simulink model "fft32kpt_ssr32_float"  (R2024a)
settings: Solver=VariableStepAuto  StartTime=0.0  StopTime=sample_period*N*6  RelTol=1e-3
PreLoadFcn:
  | clk_freq = 570e6;
  | SSR=32; % transpose block SSR settings...
  | sample_period = 1/(SSR*clk_freq);
  | N=32768; % fft point size
  | binw=(1/sample_period) / (2*N); % bin width
  | bin_freq = 2*pi*3*binw+pi*binw; % sin, cos freq centered in channel
  | 
  | % for transpose block
  | DATA_WIDTH=32;
  | M=32;
  | N1=N/M;
  | MEM_STYLE=4; % MEM OPTIONS: 4 - ULTRA, 0 - AUTO, 1 - BRAM, 5 - MIXED
InitFcn:
  | clk_freq = 570e6;
  | SSR=32; % transpose block SSR settings...
  | sample_period = 1/(SSR*clk_freq);
  | N=32768; % fft point size
  | binw=(1/sample_period) / (2*N); % bin width
  | bin_freq = 2*pi*3*binw+pi*binw; % sin, cos freq centered in channel
  | 
  | % for transpose block
  | DATA_WIDTH=32;
  | M=32;
  | N1=N/M;
  | MEM_STYLE=4; % MEM OPTIONS: 4 - ULTRA, 0 - AUTO, 1 - BRAM, 5 - MIXED
undefined symbols (not defined in the file or in its folder): None, S, vsva2197, xcvc1902
libraries: hdlBasic x139, aieBasic x95, aieUtilities x32, aieDSP x32, hdlUtilities x32, matrix_library x32, hdlSSR x12, hdlDSPIP x1, simulink x1, dspxfrm3 x1, vmcUtilities x1
(part 3 of 4)

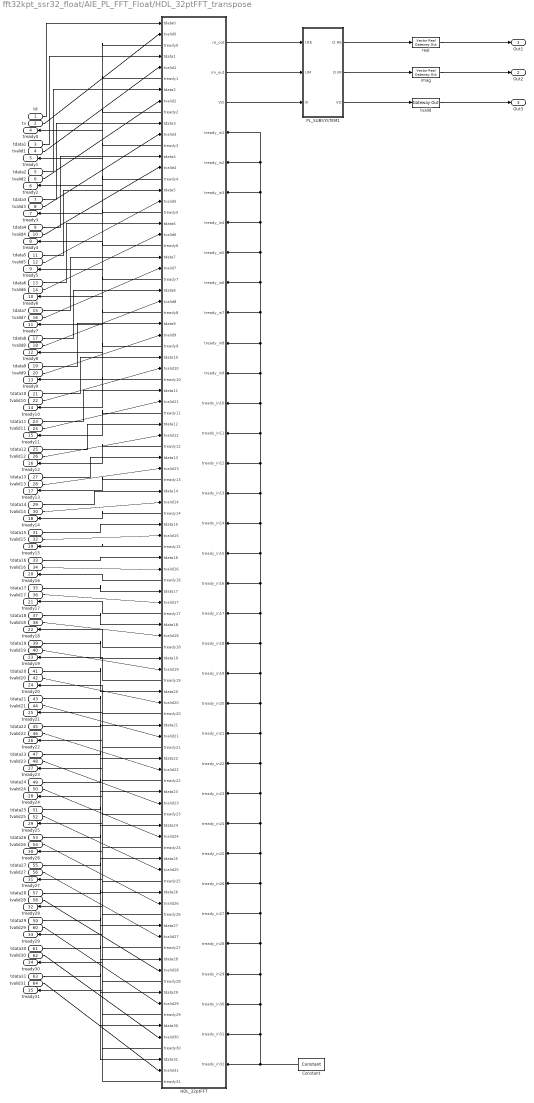
== system fft32kpt_ssr32_float/AIE_PL_FFT_Float/HDL_32ptFFT_transpose ==
  td : Inport
  tv : Inport  Port=2
  tdata1 : Inport  Port=3
  tvalid1 : Inport  Port=4
  tdata2 : Inport  Port=5
  tvalid2 : Inport  Port=6
  tdata3 : Inport  Port=7
  tvalid3 : Inport  Port=8
  tdata4 : Inport  Port=9
  tvalid4 : Inport  Port=10
  tdata5 : Inport  Port=11
  tvalid5 : Inport  Port=12
  tdata6 : Inport  Port=13
  tvalid6 : Inport  Port=14
  tdata7 : Inport  Port=15
  tvalid7 : Inport  Port=16
  tdata8 : Inport  Port=17
  tvalid8 : Inport  Port=18
  tdata9 : Inport  Port=19
  tvalid9 : Inport  Port=20
  tdata10 : Inport  Port=21
  tvalid10 : Inport  Port=22
  tdata11 : Inport  Port=23
  tvalid11 : Inport  Port=24
  tdata12 : Inport  Port=25
  tvalid12 : Inport  Port=26
  tdata13 : Inport  Port=27
  tvalid13 : Inport  Port=28
  tdata14 : Inport  Port=29
  tvalid14 : Inport  Port=30
  tdata15 : Inport  Port=31
  tvalid15 : Inport  Port=32
  tdata16 : Inport  Port=33
  tvalid16 : Inport  Port=34
  tdata17 : Inport  Port=35
  tvalid17 : Inport  Port=36
  tdata18 : Inport  Port=37
  tvalid18 : Inport  Port=38
  tdata19 : Inport  Port=39
  tvalid19 : Inport  Port=40
  tdata20 : Inport  Port=41
  tvalid20 : Inport  Port=42
  tdata21 : Inport  Port=43
  tvalid21 : Inport  Port=44
  tdata22 : Inport  Port=45
  tvalid22 : Inport  Port=46
  tdata23 : Inport  Port=47
  tvalid23 : Inport  Port=48
  tdata24 : Inport  Port=49
  tvalid24 : Inport  Port=50
  tdata25 : Inport  Port=51
  tvalid25 : Inport  Port=52
  tdata26 : Inport  Port=53
  tvalid26 : Inport  Port=54
  tdata27 : Inport  Port=55
  tvalid27 : Inport  Port=56
  tdata28 : Inport  Port=57
  tvalid28 : Inport  Port=58
  tdata29 : Inport  Port=59
  tvalid29 : Inport  Port=60
  tdata30 : Inport  Port=61
  tvalid30 : Inport  Port=62
  tdata31 : Inport  Port=63
  tvalid31 : Inport  Port=64
  Constant : hdlBasic/Constant  const=1.0  gui_display_data_type=Boolean  arith_type=Boolean  n_bits=16  bin_pt=14  preci_type=Single  exp_width=8  frac_width=24  explicit_period=on  period=1/clk_freq  XmcBlockStatus=1  maskContainerNames=tabcontainer1  block_type=constant  block_config=sysgen:Constant_config
  HDL_32ptFFT : Subsystem
      settings: PortSchema="{\"entries\":[{\"content\":{\"sides\":[{\"content\":{\"connectorIds\":[\"In1\",\"In2\",\"Out4\",\"In3\",\"In4\",\"Out5\",\"In5\",\"In6\",\"Out6\",\"In7\",\"In8\",\"Out7\",\"In9\",\"In10\",\"Out8\",\"In11\",\"In12\",\"Out9\",\"In13\",\"In14\",\"Out10\",\"In15\",\"In16\",\"Out11\",\"In17\",\"In18\",\"Out12\",\"In19\",\"In20\",\"Out13\",\"In21\",\"In22\",\"Out14\",\"In23\",\"In24\",\"Out15\",\"In25\",\"In26\",\"Out16\",\"In27\",\"In28\",\"Out17\",\"In29\",\"In30\",\"Out18\",\"In31\",\"In32\",\"Out19\",\"In33\",\"In34\",\"Out20\",\"In35\",\"In36\",\"Out21\",\"In37\",\"In38\",\"Out22\",\"In39\",\"In40\",\"Out23\",\"In41\",\"In42\",\"Out24\",\"In43\",\"In44\",\"Out25\",\"In45\",\"In46\",\"Out26\",\"In47\",\"In48\",\"Out27\",\"In49\",\"In50\",\"Out28\",\"In51\",\"In52\",\"Out29\",\"In53\",\"In54\",\"Out30\",\"In55\",\"In56\",\"Out31\",\"In57\",\"In58\",\"Out32\",\"In59\",\"In60\",\"Out33\",\"In61\",\"In62\",\"Out34\",\"In63\",\"In64\",\"Out35\"]},\"type\":\"ConnectorPlacement.EquallySpacedRectSide\",\"uuid\":\"a3725b6b-e4a3-4f45-ab24-220566ddd85d\"},{\"content\":{\"connectorIds\":[\"Out1\",\"Out2\",\"Out3\",\"In65\",\"In66\",\"In67\",\"In68\",\"In69\",\"In70\",\"In71\",\"In72\",\"In73\",\"In74\",\"In75\",\"In76\",\"In77\",\"In78\",\"In79\",\"In80\",\"In81\",\"In82\",\"In83\",\"In84\",\"In85\",\"In86\",\"In87\",\"In88\",\"In89\",\"In90\",\"In91\",\"In92\",\"In93\",\"In94\",\"In95\",\"In96\"],\"side\":\"RIGHT\"},\"type\":\"ConnectorPlacement.EquallySpacedRectSide\",\"uuid\":\"6d1cacb8-7866-41d1-bf7d-cacacc53b5ea\"},{\"content\":{\"side\":\"TOP\"},\"type\":\"ConnectorPlacement.EquallySpacedRectSide\",\"uuid\":\"e352e270-c6f1-4bf3-b401-eafc9b9ac14e\"},{\"content\":{\"side\":\"BOTTOM\"},\"type\":\"ConnectorPlacement.EquallySpacedRectSide\",\"uuid\":\"85cad029-9e0a-42ad-b7dd-28c8d75053c6\"}]},\"type\":\"ConnectorPlacement.EquallySpacedConnector\",\"uuid\":\"92e4a087-3b5f-44ab-84c8-8a9b01a0fbf2\"}],\"packageUris\":[\"http://schema.mathworks.com/mf0/Connector/R2020b\"],\"version\":\"1.0\"}"
  PL_SUBSYSTEM1 : Subsystem
  imag : hdlSSR/Vector Real Gateway Out  inherit_from_input=on  hdl_port=on  sg_ssr=32  rows=1  columns=1  UseAsDAC=off  DACChannel='1'  interface=None  automatic_assignment=on  address_offset=hex2dec('00')  intf_name=''  intf_description=''  timing_constraint=None  locs_specified=off  LOCs={}  io_standard={}  block_type=realgatewayout_ssr  XmcBlockStatus=1  sg_ssr_prev=32  maskContainerNames=group4  block_width_w=590  block_height_w=620  block_width=620  block_height=750
  real : hdlSSR/Vector Real Gateway Out  inherit_from_input=on  hdl_port=on  sg_ssr=32  rows=1  columns=1  UseAsDAC=off  DACChannel='1'  interface=None  automatic_assignment=on  address_offset=hex2dec('00')  intf_name=''  intf_description=''  timing_constraint=None  locs_specified=off  LOCs={}  io_standard={}  block_type=realgatewayout_ssr  XmcBlockStatus=1  sg_ssr_prev=32  maskContainerNames=group4  block_width_w=590  block_height_w=620  block_width=620  block_height=750
  tvalid : hdlBasic/Gateway Out  inherit_from_input=on  bool_to_boolean=off  hdl_port=on  rows=1  columns=1  UseAsDAC=off  DACChannel='1'  interface=None  automatic_assignment=on  address_offset=hex2dec('00')  intf_name=''  intf_description=''  timing_constraint=None  locs_specified=off  LOCs={}  io_standard={}  XmcBlockStatus=1  maskContainerNames=group4  block_type=gatewayout  block_config=sysgen:gateway_out_config  block_width_w=590  block_height_w=620  block_width=620  block_height=750
  Out1 : Outport
  Out2 : Outport  Port=2
  Out3 : Outport  Port=3
  tready0 : Outport  Port=4
  tready1 : Outport  Port=5
  tready2 : Outport  Port=6
  tready3 : Outport  Port=7
  tready4 : Outport  Port=8
  tready5 : Outport  Port=9
  tready6 : Outport  Port=10
  tready7 : Outport  Port=11
  tready8 : Outport  Port=12
  tready9 : Outport  Port=13
  tready10 : Outport  Port=14
  tready11 : Outport  Port=15
  tready12 : Outport  Port=16
  tready13 : Outport  Port=17
  tready14 : Outport  Port=18
  tready15 : Outport  Port=19
  tready16 : Outport  Port=20
  tready17 : Outport  Port=21
  tready18 : Outport  Port=22
  tready19 : Outport  Port=23
  tready20 : Outport  Port=24
  tready21 : Outport  Port=25
  tready22 : Outport  Port=26
  tready23 : Outport  Port=27
  tready24 : Outport  Port=28
  tready25 : Outport  Port=29
  tready26 : Outport  Port=30
  tready27 : Outport  Port=31
  tready28 : Outport  Port=32
  tready29 : Outport  Port=33
  tready30 : Outport  Port=34
  tready31 : Outport  Port=35
  wires:
  HDL_32ptFFT/16(tready12) -> tready12/1
  tdata23/1 -> HDL_32ptFFT/47(tdata23)
  tdata17/1 -> HDL_32ptFFT/35(tdata17)
  HDL_32ptFFT/22(tready18) -> tready18/1
  tdata6/1 -> HDL_32ptFFT/13(tdata6)
  HDL_32ptFFT/17(tready13) -> tready13/1
  tvalid26/1 -> HDL_32ptFFT/54(tvalid26)
  HDL_32ptFFT/8(tready4) -> tready4/1
  tv/1 -> HDL_32ptFFT/2(tvalid0)
  HDL_32ptFFT/31(tready27) -> tready27/1
  tvalid11/1 -> HDL_32ptFFT/24(tvalid11)
  real/1 -> Out1/1
  tvalid27/1 -> HDL_32ptFFT/56(tvalid27)
  HDL_32ptFFT/34(tready30) -> tready30/1
  tdata10/1 -> HDL_32ptFFT/21(tdata10)
  tvalid6/1 -> HDL_32ptFFT/14(tvalid6)
  HDL_32ptFFT/5(tready1) -> tready1/1
  tvalid3/1 -> HDL_32ptFFT/8(tvalid3)
  tvalid22/1 -> HDL_32ptFFT/46(tvalid22)
  HDL_32ptFFT/32(tready28) -> tready28/1
  tvalid4/1 -> HDL_32ptFFT/10(tvalid4)
  HDL_32ptFFT/30(tready26) -> tready26/1
  tdata1/1 -> HDL_32ptFFT/3(tdata1)
  tdata28/1 -> HDL_32ptFFT/57(tdata28)
  tdata5/1 -> HDL_32ptFFT/11(tdata5)
  HDL_32ptFFT/12(tready8) -> tready8/1
  HDL_32ptFFT/15(tready11) -> tready11/1
  tvalid31/1 -> HDL_32ptFFT/64(tvalid31)
  tdata25/1 -> HDL_32ptFFT/51(tdata25)
  tvalid25/1 -> HDL_32ptFFT/52(tvalid25)
  tvalid29/1 -> HDL_32ptFFT/60(tvalid29)
  HDL_32ptFFT/35(tready31) -> tready31/1
  tvalid2/1 -> HDL_32ptFFT/6(tvalid2)
  HDL_32ptFFT/28(tready24) -> tready24/1
  HDL_32ptFFT/13(tready9) -> tready9/1
  PL_SUBSYSTEM1/1(O.RE) -> real/1
  HDL_32ptFFT/18(tready14) -> tready14/1
  tdata27/1 -> HDL_32ptFFT/55(tdata27)
  tdata16/1 -> HDL_32ptFFT/33(tdata16)
  tdata12/1 -> HDL_32ptFFT/25(tdata12)
  tvalid18/1 -> HDL_32ptFFT/38(tvalid18)
  tdata4/1 -> HDL_32ptFFT/9(tdata4)
  tvalid16/1 -> HDL_32ptFFT/34(tvalid16)
  tdata13/1 -> HDL_32ptFFT/27(tdata13)
  imag/1 -> Out2/1
  HDL_32ptFFT/4(tready0) -> tready0/1
  tvalid28/1 -> HDL_32ptFFT/58(tvalid28)
  HDL_32ptFFT/9(tready5) -> tready5/1
  tdata18/1 -> HDL_32ptFFT/37(tdata18)
  HDL_32ptFFT/21(tready17) -> tready17/1
  tdata26/1 -> HDL_32ptFFT/53(tdata26)
  HDL_32ptFFT/6(tready2) -> tready2/1
  tdata29/1 -> HDL_32ptFFT/59(tdata29)
  tdata15/1 -> HDL_32ptFFT/31(tdata15)
  tdata11/1 -> HDL_32ptFFT/23(tdata11)
  Constant/1 -> HDL_32ptFFT/94(tready_in30), HDL_32ptFFT/93(tready_in29), HDL_32ptFFT/92(tready_in28), HDL_32ptFFT/91(tready_in27), HDL_32ptFFT/90(tready_in26), HDL_32ptFFT/89(tready_in25), HDL_32ptFFT/88(tready_in24), HDL_32ptFFT/87(tready_in23), HDL_32ptFFT/86(tready_in22), HDL_32ptFFT/85(tready_in21), HDL_32ptFFT/84(tready_in20), HDL_32ptFFT/83(tready_in19), HDL_32ptFFT/82(tready_in18), HDL_32ptFFT/81(tready_in17), HDL_32ptFFT/80(tready_in16), HDL_32ptFFT/79(tready_in15), HDL_32ptFFT/78(tready_in14), HDL_32ptFFT/77(tready_in13), HDL_32ptFFT/76(tready_in12), HDL_32ptFFT/75(tready_in11), HDL_32ptFFT/74(tready_in10), HDL_32ptFFT/73(tready_in9), HDL_32ptFFT/72(tready_in8), HDL_32ptFFT/71(tready_in7), HDL_32ptFFT/69(tready_in5), HDL_32ptFFT/68(tready_in4), HDL_32ptFFT/67(tready_in3), HDL_32ptFFT/66(tready_in2), HDL_32ptFFT/65(tready_in1), HDL_32ptFFT/70(tready_in6), HDL_32ptFFT/95(tready_in31), HDL_32ptFFT/96(tready_in32)
  tvalid23/1 -> HDL_32ptFFT/48(tvalid23)
  HDL_32ptFFT/19(tready15) -> tready15/1
  tdata19/1 -> HDL_32ptFFT/39(tdata19)
  tvalid14/1 -> HDL_32ptFFT/30(tvalid14)
  HDL_32ptFFT/10(tready6) -> tready6/1
  HDL_32ptFFT/23(tready19) -> tready19/1
  tvalid1/1 -> HDL_32ptFFT/4(tvalid1)
  tvalid10/1 -> HDL_32ptFFT/22(tvalid10)
  HDL_32ptFFT/27(tready23) -> tready23/1
  tdata9/1 -> HDL_32ptFFT/19(tdata9)
  tvalid12/1 -> HDL_32ptFFT/26(tvalid12)
  tvalid13/1 -> HDL_32ptFFT/28(tvalid13)
  HDL_32ptFFT/7(tready3) -> tready3/1
  tvalid21/1 -> HDL_32ptFFT/44(tvalid21)
  tvalid15/1 -> HDL_32ptFFT/32(tvalid15)
  tdata8/1 -> HDL_32ptFFT/17(tdata8)
  tdata20/1 -> HDL_32ptFFT/41(tdata20)
  tdata24/1 -> HDL_32ptFFT/49(tdata24)
  tvalid24/1 -> HDL_32ptFFT/50(tvalid24)
  PL_SUBSYSTEM1/3(VO) -> tvalid/1
  tvalid20/1 -> HDL_32ptFFT/42(tvalid20)
  tdata21/1 -> HDL_32ptFFT/43(tdata21)
  tdata30/1 -> HDL_32ptFFT/61(tdata30)
  tdata2/1 -> HDL_32ptFFT/5(tdata2)
  HDL_32ptFFT/11(tready7) -> tready7/1
  HDL_32ptFFT/33(tready29) -> tready29/1
  HDL_32ptFFT/24(tready20) -> tready20/1
  HDL_32ptFFT/25(tready21) -> tready21/1
  tdata3/1 -> HDL_32ptFFT/7(tdata3)
  tvalid19/1 -> HDL_32ptFFT/40(tvalid19)
  tdata31/1 -> HDL_32ptFFT/63(tdata31)
  tdata14/1 -> HDL_32ptFFT/29(tdata14)
  HDL_32ptFFT/20(tready16) -> tready16/1
  HDL_32ptFFT/3(VO) -> PL_SUBSYSTEM1/3(VI)
  HDL_32ptFFT/1(re_out) -> PL_SUBSYSTEM1/1(I.RE)
  tdata7/1 -> HDL_32ptFFT/15(tdata7)
  tvalid/1 -> Out3/1
  HDL_32ptFFT/26(tready22) -> tready22/1
  tvalid8/1 -> HDL_32ptFFT/18(tvalid8)
  HDL_32ptFFT/29(tready25) -> tready25/1
  PL_SUBSYSTEM1/2(O.IM) -> imag/1
  HDL_32ptFFT/14(tready10) -> tready10/1
  HDL_32ptFFT/2(im_out) -> PL_SUBSYSTEM1/2(I.IM)
  tdata22/1 -> HDL_32ptFFT/45(tdata22)
  tvalid5/1 -> HDL_32ptFFT/12(tvalid5)
  tvalid30/1 -> HDL_32ptFFT/62(tvalid30)
  tvalid7/1 -> HDL_32ptFFT/16(tvalid7)
  td/1 -> HDL_32ptFFT/1(tdata0)
  tvalid17/1 -> HDL_32ptFFT/36(tvalid17)
  tvalid9/1 -> HDL_32ptFFT/20(tvalid9)

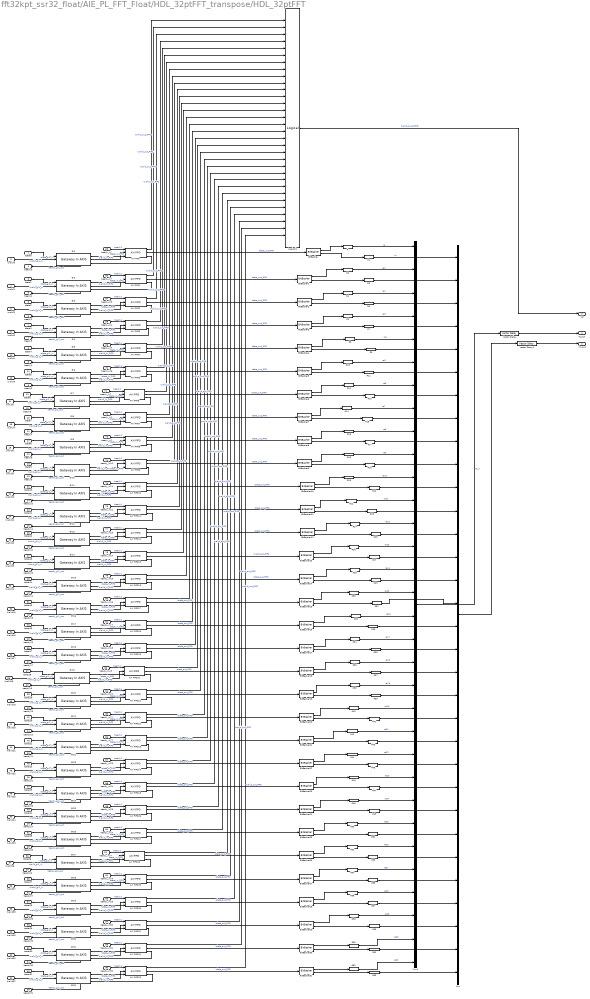
== system fft32kpt_ssr32_float/AIE_PL_FFT_Float/HDL_32ptFFT_transpose/HDL_32ptFFT ==
  tdata0 : Inport
  tvalid0 : Inport  Port=2
  tdata1 : Inport  Port=3
  tvalid1 : Inport  Port=4
  tdata2 : Inport  Port=5
  tvalid2 : Inport  Port=6
  tdata3 : Inport  Port=7
  tvalid3 : Inport  Port=8
  tdata4 : Inport  Port=9
  tvalid4 : Inport  Port=10
  tdata5 : Inport  Port=11
  tvalid5 : Inport  Port=12
  tdata6 : Inport  Port=13
  tvalid6 : Inport  Port=14
  tdata7 : Inport  Port=15
  tvalid7 : Inport  Port=16
  tdata8 : Inport  Port=17
  tvalid8 : Inport  Port=18
  tdata9 : Inport  Port=19
  tvalid9 : Inport  Port=20
  tdata10 : Inport  Port=21
  tvalid10 : Inport  Port=22
  tdata11 : Inport  Port=23
  tvalid11 : Inport  Port=24
  tdata12 : Inport  Port=25
  tvalid12 : Inport  Port=26
  tdata13 : Inport  Port=27
  tvalid13 : Inport  Port=28
  tdata14 : Inport  Port=29
  tvalid14 : Inport  Port=30
  tdata15 : Inport  Port=31
  tvalid15 : Inport  Port=32
  tdata16 : Inport  Port=33
  tvalid16 : Inport  Port=34
  tdata17 : Inport  Port=35
  tvalid17 : Inport  Port=36
  tdata18 : Inport  Port=37
  tvalid18 : Inport  Port=38
  tdata19 : Inport  Port=39
  tvalid19 : Inport  Port=40
  tdata20 : Inport  Port=41
  tvalid20 : Inport  Port=42
  tdata21 : Inport  Port=43
  tvalid21 : Inport  Port=44
  tdata22 : Inport  Port=45
  tvalid22 : Inport  Port=46
  tdata23 : Inport  Port=47
  tvalid23 : Inport  Port=48
  tdata24 : Inport  Port=49
  tvalid24 : Inport  Port=50
  tdata25 : Inport  Port=51
  tvalid25 : Inport  Port=52
  tdata26 : Inport  Port=53
  tvalid26 : Inport  Port=54
  tdata27 : Inport  Port=55
  tvalid27 : Inport  Port=56
  tdata28 : Inport  Port=57
  tvalid28 : Inport  Port=58
  tdata29 : Inport  Port=59
  tvalid29 : Inport  Port=60
  tdata30 : Inport  Port=61
  tvalid30 : Inport  Port=62
  tdata31 : Inport  Port=63
  tvalid31 : Inport  Port=64
  tready_in1 : Inport  Port=65
  tready_in2 : Inport  Port=66
  tready_in3 : Inport  Port=67
  tready_in4 : Inport  Port=68
  tready_in5 : Inport  Port=69
  tready_in6 : Inport  Port=70
  tready_in7 : Inport  Port=71
  tready_in8 : Inport  Port=72
  tready_in9 : Inport  Port=73
  tready_in10 : Inport  Port=74
  tready_in11 : Inport  Port=75
  tready_in12 : Inport  Port=76
  tready_in13 : Inport  Port=77
  tready_in14 : Inport  Port=78
  tready_in15 : Inport  Port=79
  tready_in16 : Inport  Port=80
  tready_in17 : Inport  Port=81
  tready_in18 : Inport  Port=82
  tready_in19 : Inport  Port=83
  tready_in20 : Inport  Port=84
  tready_in21 : Inport  Port=85
  tready_in22 : Inport  Port=86
  tready_in23 : Inport  Port=87
  tready_in24 : Inport  Port=88
  tready_in25 : Inport  Port=89
  tready_in26 : Inport  Port=90
  tready_in27 : Inport  Port=91
  tready_in28 : Inport  Port=92
  tready_in29 : Inport  Port=93
  tready_in30 : Inport  Port=94
  tready_in31 : Inport  Port=95
  tready_in32 : Inport  Port=96
  AXI FIFO{,1..31} (32 alike) : hdlBasic/AXI FIFO  input_depth_axis=128  actual_fifo_depth_label=130  enable_tdata=on  enable_tdest=off  enable_tstrb=off  enable_tready=on  enable_tid=off  enable_tuser=off  enable_tkeep=off  enable_tlast=off  has_aresetn=off  enable_data_counts_axis=off  fifo_implementation_type_axis=Common Clock Block RAM  trim_axipin_name=on  programmable_full_type_axis=Full  full_threshold_assert_value_axis=0  programmable_empty_type_axis=Empty  empty_threshold_assert_value_axis=1022  underflow_flag_axi=0  underflow_sense_axi=Active High  overflow_flag_axi=0  overflow_sense_axi=Active High  simulation_type=fast_sim  XmcBlockStatus=1  maskContainerNames=tabcontainer1  block_type=axi_fifo  block_config=sysgen:AXI_FIFO_config
  BitBasher : hdlBasic/BitBasher  bitexpr=|  display_expr=off  sr_1=re  arith_type1=Unsigned  bin_pt1=0  sr_2=im  arith_type2=Unsigned  bin_pt2=0  sr_3=3  arith_type3=Unsigned  bin_pt3=0  sr_4=4  arith_type4=Unsigned  bin_pt4=0  XmcBlockStatus=1  maskContainerNames=group1  block_type=bitbasher  block_config=sysgen:BitBasher_config
      | re={inp[31:0]};
      | im={inp[63:32]};
  BitBasher1 : hdlBasic/BitBasher  bitexpr=|  display_expr=off  sr_1=re  arith_type1=Unsigned  bin_pt1=0  sr_2=im  arith_type2=Unsigned  bin_pt2=0  sr_3=3  arith_type3=Unsigned  bin_pt3=0  sr_4=4  arith_type4=Unsigned  bin_pt4=0  XmcBlockStatus=1  maskContainerNames=group1  block_type=bitbasher  block_config=sysgen:BitBasher_config
      | re={inp[31:0]};
      | im={inp[63:32]};
  BitBasher10 : hdlBasic/BitBasher  bitexpr=|  display_expr=off  sr_1=re  arith_type1=Unsigned  bin_pt1=0  sr_2=im  arith_type2=Unsigned  bin_pt2=0  sr_3=3  arith_type3=Unsigned  bin_pt3=0  sr_4=4  arith_type4=Unsigned  bin_pt4=0  XmcBlockStatus=1  maskContainerNames=group1  block_type=bitbasher  block_config=sysgen:BitBasher_config
      | re={inp[31:0]};
      | im={inp[63:32]};
  BitBasher11 : hdlBasic/BitBasher  bitexpr=|  display_expr=off  sr_1=re  arith_type1=Unsigned  bin_pt1=0  sr_2=im  arith_type2=Unsigned  bin_pt2=0  sr_3=3  arith_type3=Unsigned  bin_pt3=0  sr_4=4  arith_type4=Unsigned  bin_pt4=0  XmcBlockStatus=1  maskContainerNames=group1  block_type=bitbasher  block_config=sysgen:BitBasher_config
      | re={inp[31:0]};
      | im={inp[63:32]};
  BitBasher12 : hdlBasic/BitBasher  bitexpr=|  display_expr=off  sr_1=re  arith_type1=Unsigned  bin_pt1=0  sr_2=im  arith_type2=Unsigned  bin_pt2=0  sr_3=3  arith_type3=Unsigned  bin_pt3=0  sr_4=4  arith_type4=Unsigned  bin_pt4=0  XmcBlockStatus=1  maskContainerNames=group1  block_type=bitbasher  block_config=sysgen:BitBasher_config
      | re={inp[31:0]};
      | im={inp[63:32]};
  BitBasher13 : hdlBasic/BitBasher  bitexpr=|  display_expr=off  sr_1=re  arith_type1=Unsigned  bin_pt1=0  sr_2=im  arith_type2=Unsigned  bin_pt2=0  sr_3=3  arith_type3=Unsigned  bin_pt3=0  sr_4=4  arith_type4=Unsigned  bin_pt4=0  XmcBlockStatus=1  maskContainerNames=group1  block_type=bitbasher  block_config=sysgen:BitBasher_config
      | re={inp[31:0]};
      | im={inp[63:32]};
  BitBasher14 : hdlBasic/BitBasher  bitexpr=|  display_expr=off  sr_1=re  arith_type1=Unsigned  bin_pt1=0  sr_2=im  arith_type2=Unsigned  bin_pt2=0  sr_3=3  arith_type3=Unsigned  bin_pt3=0  sr_4=4  arith_type4=Unsigned  bin_pt4=0  XmcBlockStatus=1  maskContainerNames=group1  block_type=bitbasher  block_config=sysgen:BitBasher_config
      | re={inp[31:0]};
      | im={inp[63:32]};
  BitBasher15 : hdlBasic/BitBasher  bitexpr=|  display_expr=off  sr_1=re  arith_type1=Unsigned  bin_pt1=0  sr_2=im  arith_type2=Unsigned  bin_pt2=0  sr_3=3  arith_type3=Unsigned  bin_pt3=0  sr_4=4  arith_type4=Unsigned  bin_pt4=0  XmcBlockStatus=1  maskContainerNames=group1  block_type=bitbasher  block_config=sysgen:BitBasher_config
      | re={inp[31:0]};
      | im={inp[63:32]};
  BitBasher16 : hdlBasic/BitBasher  bitexpr=|  display_expr=off  sr_1=re  arith_type1=Unsigned  bin_pt1=0  sr_2=im  arith_type2=Unsigned  bin_pt2=0  sr_3=3  arith_type3=Unsigned  bin_pt3=0  sr_4=4  arith_type4=Unsigned  bin_pt4=0  XmcBlockStatus=1  maskContainerNames=group1  block_type=bitbasher  block_config=sysgen:BitBasher_config
      | re={inp[31:0]};
      | im={inp[63:32]};
  BitBasher17 : hdlBasic/BitBasher  bitexpr=|  display_expr=off  sr_1=re  arith_type1=Unsigned  bin_pt1=0  sr_2=im  arith_type2=Unsigned  bin_pt2=0  sr_3=3  arith_type3=Unsigned  bin_pt3=0  sr_4=4  arith_type4=Unsigned  bin_pt4=0  XmcBlockStatus=1  maskContainerNames=group1  block_type=bitbasher  block_config=sysgen:BitBasher_config
      | re={inp[31:0]};
      | im={inp[63:32]};
  BitBasher18 : hdlBasic/BitBasher  bitexpr=|  display_expr=off  sr_1=re  arith_type1=Unsigned  bin_pt1=0  sr_2=im  arith_type2=Unsigned  bin_pt2=0  sr_3=3  arith_type3=Unsigned  bin_pt3=0  sr_4=4  arith_type4=Unsigned  bin_pt4=0  XmcBlockStatus=1  maskContainerNames=group1  block_type=bitbasher  block_config=sysgen:BitBasher_config
      | re={inp[31:0]};
      | im={inp[63:32]};
  BitBasher19 : hdlBasic/BitBasher  bitexpr=|  display_expr=off  sr_1=re  arith_type1=Unsigned  bin_pt1=0  sr_2=im  arith_type2=Unsigned  bin_pt2=0  sr_3=3  arith_type3=Unsigned  bin_pt3=0  sr_4=4  arith_type4=Unsigned  bin_pt4=0  XmcBlockStatus=1  maskContainerNames=group1  block_type=bitbasher  block_config=sysgen:BitBasher_config
      | re={inp[31:0]};
      | im={inp[63:32]};
  BitBasher2 : hdlBasic/BitBasher  bitexpr=|  display_expr=off  sr_1=re  arith_type1=Unsigned  bin_pt1=0  sr_2=im  arith_type2=Unsigned  bin_pt2=0  sr_3=3  arith_type3=Unsigned  bin_pt3=0  sr_4=4  arith_type4=Unsigned  bin_pt4=0  XmcBlockStatus=1  maskContainerNames=group1  block_type=bitbasher  block_config=sysgen:BitBasher_config
      | re={inp[31:0]};
      | im={inp[63:32]};
  BitBasher20 : hdlBasic/BitBasher  bitexpr=|  display_expr=off  sr_1=re  arith_type1=Unsigned  bin_pt1=0  sr_2=im  arith_type2=Unsigned  bin_pt2=0  sr_3=3  arith_type3=Unsigned  bin_pt3=0  sr_4=4  arith_type4=Unsigned  bin_pt4=0  XmcBlockStatus=1  maskContainerNames=group1  block_type=bitbasher  block_config=sysgen:BitBasher_config
      | re={inp[31:0]};
      | im={inp[63:32]};
  BitBasher21 : hdlBasic/BitBasher  bitexpr=|  display_expr=off  sr_1=re  arith_type1=Unsigned  bin_pt1=0  sr_2=im  arith_type2=Unsigned  bin_pt2=0  sr_3=3  arith_type3=Unsigned  bin_pt3=0  sr_4=4  arith_type4=Unsigned  bin_pt4=0  XmcBlockStatus=1  maskContainerNames=group1  block_type=bitbasher  block_config=sysgen:BitBasher_config
      | re={inp[31:0]};
      | im={inp[63:32]};
  BitBasher22 : hdlBasic/BitBasher  bitexpr=|  display_expr=off  sr_1=re  arith_type1=Unsigned  bin_pt1=0  sr_2=im  arith_type2=Unsigned  bin_pt2=0  sr_3=3  arith_type3=Unsigned  bin_pt3=0  sr_4=4  arith_type4=Unsigned  bin_pt4=0  XmcBlockStatus=1  maskContainerNames=group1  block_type=bitbasher  block_config=sysgen:BitBasher_config
      | re={inp[31:0]};
      | im={inp[63:32]};
  BitBasher23 : hdlBasic/BitBasher  bitexpr=|  display_expr=off  sr_1=re  arith_type1=Unsigned  bin_pt1=0  sr_2=im  arith_type2=Unsigned  bin_pt2=0  sr_3=3  arith_type3=Unsigned  bin_pt3=0  sr_4=4  arith_type4=Unsigned  bin_pt4=0  XmcBlockStatus=1  maskContainerNames=group1  block_type=bitbasher  block_config=sysgen:BitBasher_config
      | re={inp[31:0]};
      | im={inp[63:32]};
  BitBasher24 : hdlBasic/BitBasher  bitexpr=|  display_expr=off  sr_1=re  arith_type1=Unsigned  bin_pt1=0  sr_2=im  arith_type2=Unsigned  bin_pt2=0  sr_3=3  arith_type3=Unsigned  bin_pt3=0  sr_4=4  arith_type4=Unsigned  bin_pt4=0  XmcBlockStatus=1  maskContainerNames=group1  block_type=bitbasher  block_config=sysgen:BitBasher_config
      | re={inp[31:0]};
      | im={inp[63:32]};
  BitBasher25 : hdlBasic/BitBasher  bitexpr=|  display_expr=off  sr_1=re  arith_type1=Unsigned  bin_pt1=0  sr_2=im  arith_type2=Unsigned  bin_pt2=0  sr_3=3  arith_type3=Unsigned  bin_pt3=0  sr_4=4  arith_type4=Unsigned  bin_pt4=0  XmcBlockStatus=1  maskContainerNames=group1  block_type=bitbasher  block_config=sysgen:BitBasher_config
      | re={inp[31:0]};
      | im={inp[63:32]};
  BitBasher26 : hdlBasic/BitBasher  bitexpr=|  display_expr=off  sr_1=re  arith_type1=Unsigned  bin_pt1=0  sr_2=im  arith_type2=Unsigned  bin_pt2=0  sr_3=3  arith_type3=Unsigned  bin_pt3=0  sr_4=4  arith_type4=Unsigned  bin_pt4=0  XmcBlockStatus=1  maskContainerNames=group1  block_type=bitbasher  block_config=sysgen:BitBasher_config
      | re={inp[31:0]};
      | im={inp[63:32]};
  BitBasher27 : hdlBasic/BitBasher  bitexpr=|  display_expr=off  sr_1=re  arith_type1=Unsigned  bin_pt1=0  sr_2=im  arith_type2=Unsigned  bin_pt2=0  sr_3=3  arith_type3=Unsigned  bin_pt3=0  sr_4=4  arith_type4=Unsigned  bin_pt4=0  XmcBlockStatus=1  maskContainerNames=group1  block_type=bitbasher  block_config=sysgen:BitBasher_config
      | re={inp[31:0]};
      | im={inp[63:32]};
  BitBasher28 : hdlBasic/BitBasher  bitexpr=|  display_expr=off  sr_1=re  arith_type1=Unsigned  bin_pt1=0  sr_2=im  arith_type2=Unsigned  bin_pt2=0  sr_3=3  arith_type3=Unsigned  bin_pt3=0  sr_4=4  arith_type4=Unsigned  bin_pt4=0  XmcBlockStatus=1  maskContainerNames=group1  block_type=bitbasher  block_config=sysgen:BitBasher_config
      | re={inp[31:0]};
      | im={inp[63:32]};
  BitBasher29 : hdlBasic/BitBasher  bitexpr=|  display_expr=off  sr_1=re  arith_type1=Unsigned  bin_pt1=0  sr_2=im  arith_type2=Unsigned  bin_pt2=0  sr_3=3  arith_type3=Unsigned  bin_pt3=0  sr_4=4  arith_type4=Unsigned  bin_pt4=0  XmcBlockStatus=1  maskContainerNames=group1  block_type=bitbasher  block_config=sysgen:BitBasher_config
      | re={inp[31:0]};
      | im={inp[63:32]};
  BitBasher3 : hdlBasic/BitBasher  bitexpr=|  display_expr=off  sr_1=re  arith_type1=Unsigned  bin_pt1=0  sr_2=im  arith_type2=Unsigned  bin_pt2=0  sr_3=3  arith_type3=Unsigned  bin_pt3=0  sr_4=4  arith_type4=Unsigned  bin_pt4=0  XmcBlockStatus=1  maskContainerNames=group1  block_type=bitbasher  block_config=sysgen:BitBasher_config
      | re={inp[31:0]};
      | im={inp[63:32]};
  BitBasher30 : hdlBasic/BitBasher  bitexpr=|  display_expr=off  sr_1=re  arith_type1=Unsigned  bin_pt1=0  sr_2=im  arith_type2=Unsigned  bin_pt2=0  sr_3=3  arith_type3=Unsigned  bin_pt3=0  sr_4=4  arith_type4=Unsigned  bin_pt4=0  XmcBlockStatus=1  maskContainerNames=group1  block_type=bitbasher  block_config=sysgen:BitBasher_config
      | re={inp[31:0]};
      | im={inp[63:32]};
  BitBasher31 : hdlBasic/BitBasher  bitexpr=|  display_expr=off  sr_1=re  arith_type1=Unsigned  bin_pt1=0  sr_2=im  arith_type2=Unsigned  bin_pt2=0  sr_3=3  arith_type3=Unsigned  bin_pt3=0  sr_4=4  arith_type4=Unsigned  bin_pt4=0  XmcBlockStatus=1  maskContainerNames=group1  block_type=bitbasher  block_config=sysgen:BitBasher_config
      | re={inp[31:0]};
      | im={inp[63:32]};
  BitBasher4 : hdlBasic/BitBasher  bitexpr=|  display_expr=off  sr_1=re  arith_type1=Unsigned  bin_pt1=0  sr_2=im  arith_type2=Unsigned  bin_pt2=0  sr_3=3  arith_type3=Unsigned  bin_pt3=0  sr_4=4  arith_type4=Unsigned  bin_pt4=0  XmcBlockStatus=1  maskContainerNames=group1  block_type=bitbasher  block_config=sysgen:BitBasher_config
      | re={inp[31:0]};
      | im={inp[63:32]};
  BitBasher5 : hdlBasic/BitBasher  bitexpr=|  display_expr=off  sr_1=re  arith_type1=Unsigned  bin_pt1=0  sr_2=im  arith_type2=Unsigned  bin_pt2=0  sr_3=3  arith_type3=Unsigned  bin_pt3=0  sr_4=4  arith_type4=Unsigned  bin_pt4=0  XmcBlockStatus=1  maskContainerNames=group1  block_type=bitbasher  block_config=sysgen:BitBasher_config
      | re={inp[31:0]};
      | im={inp[63:32]};
  BitBasher6 : hdlBasic/BitBasher  bitexpr=|  display_expr=off  sr_1=re  arith_type1=Unsigned  bin_pt1=0  sr_2=im  arith_type2=Unsigned  bin_pt2=0  sr_3=3  arith_type3=Unsigned  bin_pt3=0  sr_4=4  arith_type4=Unsigned  bin_pt4=0  XmcBlockStatus=1  maskContainerNames=group1  block_type=bitbasher  block_config=sysgen:BitBasher_config
      | re={inp[31:0]};
      | im={inp[63:32]};
  BitBasher7 : hdlBasic/BitBasher  bitexpr=|  display_expr=off  sr_1=re  arith_type1=Unsigned  bin_pt1=0  sr_2=im  arith_type2=Unsigned  bin_pt2=0  sr_3=3  arith_type3=Unsigned  bin_pt3=0  sr_4=4  arith_type4=Unsigned  bin_pt4=0  XmcBlockStatus=1  maskContainerNames=group1  block_type=bitbasher  block_config=sysgen:BitBasher_config
      | re={inp[31:0]};
      | im={inp[63:32]};
  BitBasher8 : hdlBasic/BitBasher  bitexpr=|  display_expr=off  sr_1=re  arith_type1=Unsigned  bin_pt1=0  sr_2=im  arith_type2=Unsigned  bin_pt2=0  sr_3=3  arith_type3=Unsigned  bin_pt3=0  sr_4=4  arith_type4=Unsigned  bin_pt4=0  XmcBlockStatus=1  maskContainerNames=group1  block_type=bitbasher  block_config=sysgen:BitBasher_config
      | re={inp[31:0]};
      | im={inp[63:32]};
  BitBasher9 : hdlBasic/BitBasher  bitexpr=|  display_expr=off  sr_1=re  arith_type1=Unsigned  bin_pt1=0  sr_2=im  arith_type2=Unsigned  bin_pt2=0  sr_3=3  arith_type3=Unsigned  bin_pt3=0  sr_4=4  arith_type4=Unsigned  bin_pt4=0  XmcBlockStatus=1  maskContainerNames=group1  block_type=bitbasher  block_config=sysgen:BitBasher_config
      | re={inp[31:0]};
      | im={inp[63:32]};
  GI{1..32} (32 alike) : hdlUtilities/Gateway In AXIS  gui_display_data_type=Fixed-point  arith_type=Unsigned  n_bits=64  bin_pt=0  preci_type=Single  exp_width=16  frac_width=24  quantization=Truncate  overflow=Wrap  bool_to_boolean=off  OutSampleTime=1/clk_freq  block_type=gatewayinaxi  XmcBlockStatus=1
  Logical1 : hdlBasic/Logical  logical_function=AND  inputs=32  en=off  latency=1  precision=Full  arith_type=Unsigned  n_bits=16  bin_pt=0  align_bp=on  overflow=[]  quantization=[]  XmcBlockStatus=1  maskContainerNames=tabcontainer1  block_type=logical  block_config=sysgen:Logical_config
  Mux : Mux  Inputs=32
  Mux1 : Mux  Inputs=32
  R{,1..63} (64 alike) : hdlBasic/Reinterpret  force_arith_type=on  arith_type=Floating-point  force_bin_pt=on  bin_pt=24  XmcBlockStatus=1  maskContainerNames=group1  block_type=reinterpret  block_config=sysgen:Reinterpret_config
  Vector Delay : hdlSSR/Vector Delay  rst=off  en=off  vectorize_en=off  sg_latency=1  sg_ssr=32  reg_retiming=off  block_type=delay_ssr  XmcBlockStatus=1  sg_ssr_prev=32  maskContainerNames=group1
  Vector Delay1 : hdlSSR/Vector Delay  rst=off  en=off  vectorize_en=off  sg_latency=1  sg_ssr=32  reg_retiming=off  block_type=delay_ssr  XmcBlockStatus=1  sg_ssr_prev=32  maskContainerNames=group1
  re_out : Outport
  im_out : Outport  Port=2
  VO : Outport  Port=3
  tready0 : Outport  Port=4
  tready1 : Outport  Port=5
  tready2 : Outport  Port=6
  tready3 : Outport  Port=7
  tready4 : Outport  Port=8
  tready5 : Outport  Port=9
  tready6 : Outport  Port=10
  tready7 : Outport  Port=11
  tready8 : Outport  Port=12
  tready9 : Outport  Port=13
  tready10 : Outport  Port=14
  tready11 : Outport  Port=15
  tready12 : Outport  Port=16
  tready13 : Outport  Port=17
  tready14 : Outport  Port=18
  tready15 : Outport  Port=19
  tready16 : Outport  Port=20
  tready17 : Outport  Port=21
  tready18 : Outport  Port=22
  tready19 : Outport  Port=23
  tready20 : Outport  Port=24
  tready21 : Outport  Port=25
  tready22 : Outport  Port=26
  tready23 : Outport  Port=27
  tready24 : Outport  Port=28
  tready25 : Outport  Port=29
  tready26 : Outport  Port=30
  tready27 : Outport  Port=31
  tready28 : Outport  Port=32
  tready29 : Outport  Port=33
  tready30 : Outport  Port=34
  tready31 : Outport  Port=35
  wires:
  Logical1/1 -> VO/1  "tvalid_out_of_fifo"
  BitBasher/2 -> R1/1
  BitBasher7/2 -> R15/1
  BitBasher4/2 -> R9/1
  BitBasher13/2 -> R27/1
  Mux1/1 -> Vector Delay/1  "re_in"
  BitBasher1/2 -> R3/1
  BitBasher15/2 -> R31/1
  BitBasher2/2 -> R5/1
  BitBasher14/2 -> R29/1
  BitBasher10/2 -> R21/1
  BitBasher9/2 -> R19/1
  BitBasher11/2 -> R23/1
  BitBasher3/2 -> R7/1
  BitBasher12/2 -> R25/1
  BitBasher8/2 -> R17/1
  BitBasher5/2 -> R11/1
  BitBasher6/2 -> R13/1
  BitBasher16/2 -> R33/1
  BitBasher17/2 -> R35/1
  BitBasher18/2 -> R37/1
  BitBasher19/2 -> R39/1
  BitBasher20/2 -> R41/1
  BitBasher21/2 -> R43/1
  BitBasher22/2 -> R45/1
  BitBasher23/2 -> R47/1
  BitBasher24/2 -> R49/1
  BitBasher25/2 -> R51/1
  BitBasher26/2 -> R53/1
  BitBasher27/2 -> R55/1
  BitBasher28/2 -> R57/1
  BitBasher29/2 -> R59/1
  BitBasher30/2 -> R61/1
  BitBasher31/2 -> R63/1
  BitBasher/1 -> R/1
  BitBasher1/1 -> R2/1
  BitBasher2/1 -> R4/1
  BitBasher3/1 -> R6/1
  BitBasher4/1 -> R8/1
  BitBasher5/1 -> R10/1
  BitBasher6/1 -> R12/1
  BitBasher7/1 -> R14/1
  BitBasher8/1 -> R16/1
  BitBasher9/1 -> R18/1
  BitBasher10/1 -> R20/1
  BitBasher11/1 -> R22/1
  BitBasher12/1 -> R24/1
  BitBasher13/1 -> R26/1
  BitBasher14/1 -> R28/1
  BitBasher15/1 -> R30/1
  BitBasher16/1 -> R32/1
  BitBasher17/1 -> R34/1
  BitBasher18/1 -> R36/1
  BitBasher19/1 -> R38/1
  BitBasher20/1 -> R40/1
  BitBasher21/1 -> R42/1
  BitBasher22/1 -> R44/1
  BitBasher23/1 -> R46/1
  BitBasher24/1 -> R48/1
  BitBasher25/1 -> R50/1
  BitBasher26/1 -> R52/1
  BitBasher27/1 -> R54/1
  BitBasher28/1 -> R56/1
  BitBasher29/1 -> R58/1
  BitBasher30/1 -> R60/1
  BitBasher31/1 -> R62/1
  R/1 -> Mux1/1  "re"
  R1/1 -> Mux/1  "im"
  R3/1 -> Mux/2
  R2/1 -> Mux1/2  "re1"
  R4/1 -> Mux1/3  "re2"
  R5/1 -> Mux/3
  R7/1 -> Mux/4
  R6/1 -> Mux1/4  "re3"
  R8/1 -> Mux1/5  "re4"
  R9/1 -> Mux/5
  R10/1 -> Mux1/6  "re5"
  R11/1 -> Mux/6
  R12/1 -> Mux1/7  "re6"
  R13/1 -> Mux/7
  R14/1 -> Mux1/8  "re7"
  R15/1 -> Mux/8
  R16/1 -> Mux1/9  "re8"
  R17/1 -> Mux/9
  R19/1 -> Mux/10
  R18/1 -> Mux1/10  "re9"
  R20/1 -> Mux1/11  "re10"
  R21/1 -> Mux/11
  R22/1 -> Mux1/12  "re11"
  R23/1 -> Mux/12
  R24/1 -> Mux1/13  "re12"
  R25/1 -> Mux/13
  R27/1 -> Mux/14
  R26/1 -> Mux1/14  "re13"
  R28/1 -> Mux1/15  "re14"
  R29/1 -> Mux/15
  R31/1 -> Mux/16
  R30/1 -> Mux1/16  "re15"
  R33/1 -> Mux/17
  R32/1 -> Mux1/17  "re16"
  R35/1 -> Mux/18
  R34/1 -> Mux1/18  "re17"
  R37/1 -> Mux/19
  R36/1 -> Mux1/19  "re18"
  R39/1 -> Mux/20
  R38/1 -> Mux1/20  "re19"
  R40/1 -> Mux1/21  "re20"
  R41/1 -> Mux/21
  R43/1 -> Mux/22
  R42/1 -> Mux1/22  "re21"
  R45/1 -> Mux/23
  R44/1 -> Mux1/23  "re22"
  R47/1 -> Mux/24
  R46/1 -> Mux1/24  "re23"
  R49/1 -> Mux/25
  R48/1 -> Mux1/25  "re24"
  R50/1 -> Mux1/26  "re25"
  R51/1 -> Mux/26
  R53/1 -> Mux/27
  R52/1 -> Mux1/27  "re26"
  R54/1 -> Mux1/28  "re27"
  R55/1 -> Mux/28
  R57/1 -> Mux/29
  R56/1 -> Mux1/29  "re28"
  R59/1 -> Mux/30
  R58/1 -> Mux1/30  "re29"
  R61/1 -> Mux/31
  R60/1 -> Mux1/31  "re30"
  R63/1 -> Mux/32
  R62/1 -> Mux1/32  "re31"
  Vector Delay1/1 -> im_out/1
  Mux/1 -> Vector Delay1/1
  GI1/3 -> tready0/1  "tready_gi1_out"
  tdata0/1 -> GI1/1  "tdata_gi1_in"
  tvalid0/1 -> GI1/2  "tvalid_gi1_in"
  GI1/2 -> AXI FIFO/2  "tvalid_in_FIFO"
  GI1/1 -> AXI FIFO/3  "tdata_in_FIFO"
  tready_in1/1 -> AXI FIFO/1  "tready1"
  AXI FIFO/3 -> GI1/3
  AXI FIFO/2 -> BitBasher/1  "tdata_out_FIFO"
  GI2/2 -> AXI FIFO1/2  "tvalid_in_FIFO"
  tdata1/1 -> GI2/1  "tdata_gi1_in"
  GI2/1 -> AXI FIFO1/3  "tdata_in_FIFO"
  tready_in2/1 -> AXI FIFO1/1  "tready1"
  AXI FIFO1/3 -> GI2/3
  tvalid1/1 -> GI2/2  "tvalid_gi1_in"
  GI2/3 -> tready1/1  "tready_gi1_out"
  AXI FIFO1/2 -> BitBasher1/1  "tdata_out_FIFO"
  GI3/1 -> AXI FIFO2/3  "tdata_in_FIFO"
  GI3/3 -> tready2/1  "tready_gi1_out"
  AXI FIFO2/3 -> GI3/3
  GI3/2 -> AXI FIFO2/2  "tvalid_in_FIFO"
  tdata2/1 -> GI3/1  "tdata_gi1_in"
  tvalid2/1 -> GI3/2  "tvalid_gi1_in"
  AXI FIFO2/2 -> BitBasher2/1  "tdata_out_FIFO"
  tready_in3/1 -> AXI FIFO2/1  "tready1"
  tvalid5/1 -> GI6/2  "tvalid_gi1_in"
  AXI FIFO4/3 -> GI5/3
  AXI FIFO5/3 -> GI6/3
  tready_in6/1 -> AXI FIFO5/1  "tready1"
  AXI FIFO3/3 -> GI4/3
  tready_in5/1 -> AXI FIFO4/1  "tready1"
  tdata4/1 -> GI5/1  "tdata_gi1_in"
  GI5/2 -> AXI FIFO4/2  "tvalid_in_FIFO"
  GI5/3 -> tready4/1  "tready_gi1_out"
  GI4/1 -> AXI FIFO3/3  "tdata_in_FIFO"
  GI5/1 -> AXI FIFO4/3  "tdata_in_FIFO"
  GI4/2 -> AXI FIFO3/2  "tvalid_in_FIFO"
  GI6/1 -> AXI FIFO5/3  "tdata_in_FIFO"
  tdata3/1 -> GI4/1  "tdata_gi1_in"
  tready_in4/1 -> AXI FIFO3/1  "tready1"
  tdata5/1 -> GI6/1  "tdata_gi1_in"
  tvalid4/1 -> GI5/2  "tvalid_gi1_in"
  tvalid3/1 -> GI4/2  "tvalid_gi1_in"
  GI6/3 -> tready5/1  "tready_gi1_out"
  GI6/2 -> AXI FIFO5/2  "tvalid_in_FIFO"
  GI4/3 -> tready3/1  "tready_gi1_out"
  AXI FIFO3/2 -> BitBasher3/1  "tdata_out_FIFO"
  AXI FIFO4/2 -> BitBasher4/1  "tdata_out_FIFO"
  AXI FIFO5/2 -> BitBasher5/1  "tdata_out_FIFO"
  tready_in11/1 -> AXI FIFO10/1  "tready1"
  tready_in9/1 -> AXI FIFO8/1  "tready1"
  tdata7/1 -> GI8/1  "tdata_gi1_in"
  tdata9/1 -> GI10/1  "tdata_gi1_in"
  tready_in10/1 -> AXI FIFO9/1  "tready1"
  GI12/1 -> AXI FIFO11/3  "tdata_in_FIFO"
  GI11/3 -> tready10/1  "tready_gi1_out"
  tvalid8/1 -> GI9/2  "tvalid_gi1_in"
  GI12/2 -> AXI FIFO11/2  "tvalid_in_FIFO"
  GI8/2 -> AXI FIFO7/2  "tvalid_in_FIFO"
  AXI FIFO8/3 -> GI9/3
  tready_in8/1 -> AXI FIFO7/1  "tready1"
  tvalid9/1 -> GI10/2  "tvalid_gi1_in"
  AXI FIFO7/3 -> GI8/3
  GI11/1 -> AXI FIFO10/3  "tdata_in_FIFO"
  AXI FIFO10/3 -> GI11/3
  GI10/2 -> AXI FIFO9/2  "tvalid_in_FIFO"
  GI8/3 -> tready7/1  "tready_gi1_out"
  tdata8/1 -> GI9/1  "tdata_gi1_in"
  tdata6/1 -> GI7/1  "tdata_gi1_in"
  tvalid10/1 -> GI11/2  "tvalid_gi1_in"
  GI7/2 -> AXI FIFO6/2  "tvalid_in_FIFO"
  AXI FIFO11/3 -> GI12/3
  tvalid6/1 -> GI7/2  "tvalid_gi1_in"
  GI10/1 -> AXI FIFO9/3  "tdata_in_FIFO"
  GI10/3 -> tready9/1  "tready_gi1_out"
  tvalid11/1 -> GI12/2  "tvalid_gi1_in"
  GI8/1 -> AXI FIFO7/3  "tdata_in_FIFO"
  tdata11/1 -> GI12/1  "tdata_gi1_in"
  AXI FIFO9/3 -> GI10/3
  AXI FIFO6/3 -> GI7/3
  GI7/1 -> AXI FIFO6/3  "tdata_in_FIFO"
  GI9/2 -> AXI FIFO8/2  "tvalid_in_FIFO"
  GI11/2 -> AXI FIFO10/2  "tvalid_in_FIFO"
  tdata10/1 -> GI11/1  "tdata_gi1_in"
  GI7/3 -> tready6/1  "tready_gi1_out"
  tvalid7/1 -> GI8/2  "tvalid_gi1_in"
  tready_in7/1 -> AXI FIFO6/1  "tready1"
  GI9/3 -> tready8/1  "tready_gi1_out"
  tready_in12/1 -> AXI FIFO11/1  "tready1"
  GI12/3 -> tready11/1  "tready_gi1_out"
  GI9/1 -> AXI FIFO8/3  "tdata_in_FIFO"
  AXI FIFO6/2 -> BitBasher6/1  "tdata_out_FIFO"
  AXI FIFO7/2 -> BitBasher7/1  "tdata_out_FIFO"
  AXI FIFO8/2 -> BitBasher8/1  "tdata_out_FIFO"
  AXI FIFO9/2 -> BitBasher9/1  "tdata_out_FIFO"
  AXI FIFO10/2 -> BitBasher10/1  "tdata_out_FIFO"
  AXI FIFO11/2 -> BitBasher11/1  "tdata_out_FIFO"
  tready_in18/1 -> AXI FIFO19/1  "tready1"
  GI15/3 -> tready14/1  "tready_gi1_out"
  GI22/2 -> AXI FIFO23/2  "tvalid_in_FIFO"
  AXI FIFO20/3 -> GI19/3
  tdata18/1 -> GI19/1  "tdata_gi1_in"
  GI21/2 -> AXI FIFO22/2  "tvalid_in_FIFO"
  tvalid23/1 -> GI24/2  "tvalid_gi1_in"
  tvalid13/1 -> GI14/2  "tvalid_gi1_in"
  GI20/2 -> AXI FIFO21/2  "tvalid_in_FIFO"
  tdata16/1 -> GI17/1  "tdata_gi1_in"
  GI19/1 -> AXI FIFO20/3  "tdata_in_FIFO"
  tready_in16/1 -> AXI FIFO17/1  "tready1"
  GI17/2 -> AXI FIFO18/2  "tvalid_in_FIFO"
  tdata23/1 -> GI24/1  "tdata_gi1_in"
  tready_in17/1 -> AXI FIFO18/1  "tready1"
  tvalid14/1 -> GI15/2  "tvalid_gi1_in"
  GI17/3 -> tready16/1  "tready_gi1_out"
  tvalid15/1 -> GI16/2  "tvalid_gi1_in"
  tvalid12/1 -> GI13/2  "tvalid_gi1_in"
  AXI FIFO19/3 -> GI18/3
  AXI FIFO15/3 -> GI24/3
  AXI FIFO14/3 -> GI23/3
  AXI FIFO16/3 -> GI15/3
  tready_in14/1 -> AXI FIFO13/1  "tready1"
  GI13/1 -> AXI FIFO12/3  "tdata_in_FIFO"
  GI22/3 -> tready21/1  "tready_gi1_out"
  AXI FIFO12/3 -> GI13/3
  tready_in19/1 -> AXI FIFO20/1  "tready1"
  AXI FIFO17/3 -> GI16/3
  tdata14/1 -> GI15/1  "tdata_gi1_in"
  tdata17/1 -> GI18/1  "tdata_gi1_in"
  tready_in24/1 -> AXI FIFO15/1  "tready1"
  GI14/1 -> AXI FIFO13/3  "tdata_in_FIFO"
  tvalid17/1 -> GI18/2  "tvalid_gi1_in"
  tdata21/1 -> GI22/1  "tdata_gi1_in"
  GI18/3 -> tready17/1  "tready_gi1_out"
  tready_in23/1 -> AXI FIFO14/1  "tready1"
  GI20/1 -> AXI FIFO21/3  "tdata_in_FIFO"
  GI16/3 -> tready15/1  "tready_gi1_out"
  tvalid19/1 -> GI20/2  "tvalid_gi1_in"
  GI16/1 -> AXI FIFO17/3  "tdata_in_FIFO"
  GI21/1 -> AXI FIFO22/3  "tdata_in_FIFO"
  GI13/3 -> tready12/1  "tready_gi1_out"
  AXI FIFO23/3 -> GI22/3
  GI13/2 -> AXI FIFO12/2  "tvalid_in_FIFO"
  tready_in13/1 -> AXI FIFO12/1  "tready1"
  GI19/2 -> AXI FIFO20/2  "tvalid_in_FIFO"
  GI16/2 -> AXI FIFO17/2  "tvalid_in_FIFO"
  GI18/1 -> AXI FIFO19/3  "tdata_in_FIFO"
  tvalid22/1 -> GI23/2  "tvalid_gi1_in"
  tvalid16/1 -> GI17/2  "tvalid_gi1_in"
  tdata12/1 -> GI13/1  "tdata_gi1_in"
  GI23/3 -> tready22/1  "tready_gi1_out"
  tready_in22/1 -> AXI FIFO23/1  "tready1"
  GI14/3 -> tready13/1  "tready_gi1_out"
  tvalid18/1 -> GI19/2  "tvalid_gi1_in"
  GI21/3 -> tready20/1  "tready_gi1_out"
  GI24/1 -> AXI FIFO15/3  "tdata_in_FIFO"
  tdata22/1 -> GI23/1  "tdata_gi1_in"
  GI24/3 -> tready23/1  "tready_gi1_out"
  tdata20/1 -> GI21/1  "tdata_gi1_in"
  AXI FIFO21/3 -> GI20/3
  AXI FIFO18/3 -> GI17/3
  tdata15/1 -> GI16/1  "tdata_gi1_in"
  tready_in15/1 -> AXI FIFO16/1  "tready1"
  tdata13/1 -> GI14/1  "tdata_gi1_in"
  GI17/1 -> AXI FIFO18/3  "tdata_in_FIFO"
  AXI FIFO13/3 -> GI14/3
  GI14/2 -> AXI FIFO13/2  "tvalid_in_FIFO"
  GI18/2 -> AXI FIFO19/2  "tvalid_in_FIFO"
  tready_in21/1 -> AXI FIFO22/1  "tready1"
  GI20/3 -> tready19/1  "tready_gi1_out"
  GI23/1 -> AXI FIFO14/3  "tdata_in_FIFO"
  tvalid21/1 -> GI22/2  "tvalid_gi1_in"
  AXI FIFO20/2 -> BitBasher18/1  "tdata_out_FIFO"
  tvalid20/1 -> GI21/2  "tvalid_gi1_in"
  GI15/1 -> AXI FIFO16/3  "tdata_in_FIFO"
  GI15/2 -> AXI FIFO16/2  "tvalid_in_FIFO"
  GI24/2 -> AXI FIFO15/2  "tvalid_in_FIFO"
  GI19/3 -> tready18/1  "tready_gi1_out"
  tready_in20/1 -> AXI FIFO21/1  "tready1"
  GI23/2 -> AXI FIFO14/2  "tvalid_in_FIFO"
  GI22/1 -> AXI FIFO23/3  "tdata_in_FIFO"
  AXI FIFO22/3 -> GI21/3
  tdata19/1 -> GI20/1  "tdata_gi1_in"
  AXI FIFO12/2 -> BitBasher12/1  "tdata_out_FIFO"
  AXI FIFO13/2 -> BitBasher13/1  "tvalid_out_FIFO"
  AXI FIFO16/2 -> BitBasher14/1  "tdata_out_FIFO"
  AXI FIFO17/2 -> BitBasher15/1  "tdata_out_FIFO"
  AXI FIFO18/2 -> BitBasher16/1  "tdata_out_FIFO"
  AXI FIFO19/2 -> BitBasher17/1  "tdata_out_FIFO"
  AXI FIFO21/2 -> BitBasher19/1  "tdata_out_FIFO"
  AXI FIFO22/2 -> BitBasher20/1  "tdata_out_FIFO"
  AXI FIFO23/2 -> BitBasher21/1  "tdata_out_FIFO"
  AXI FIFO14/2 -> BitBasher22/1  "tdata_out_FIFO"
  AXI FIFO15/2 -> BitBasher23/1  "tdata_out_FIFO"
  GI32/3 -> tready31/1  "tready_gi1_out"
  tdata25/1 -> GI26/1  "tdata_gi1_in"
  GI25/1 -> AXI FIFO26/3  "tdata_in_FIFO"
  GI26/2 -> AXI FIFO27/2  "tvalid_in_FIFO"
  GI32/1 -> AXI FIFO25/3  "tdata_in_FIFO"
  GI25/3 -> tready24/1  "tready_gi1_out"
  GI28/3 -> tready27/1  "tready_gi1_out"
  GI29/1 -> AXI FIFO30/3  "tdata_in_FIFO"
  GI27/2 -> AXI FIFO28/2  "tvalid_in_FIFO"
  GI28/2 -> AXI FIFO29/2  "tvalid_in_FIFO"
  GI30/1 -> AXI FIFO31/3  "tdata_in_FIFO"
  GI31/1 -> AXI FIFO24/3  "tdata_in_FIFO"
  tvalid29/1 -> GI30/2  "tvalid_gi1_in"
  GI32/2 -> AXI FIFO25/2  "tvalid_in_FIFO"
  tvalid28/1 -> GI29/2  "tvalid_gi1_in"
  AXI FIFO26/3 -> GI25/3
  tready_in29/1 -> AXI FIFO30/1  "tready1"
  GI27/3 -> tready26/1  "tready_gi1_out"
  GI29/2 -> AXI FIFO30/2  "tvalid_in_FIFO"
  tready_in32/1 -> AXI FIFO25/1  "tready1"
  tdata28/1 -> GI29/1  "tdata_gi1_in"
  tvalid31/1 -> GI32/2  "tvalid_gi1_in"
  tvalid26/1 -> GI27/2  "tvalid_gi1_in"
  tdata26/1 -> GI27/1  "tdata_gi1_in"
  tvalid30/1 -> GI31/2  "tvalid_gi1_in"
  GI30/2 -> AXI FIFO31/2  "tvalid_in_FIFO"
  GI29/3 -> tready28/1  "tready_gi1_out"
  GI31/3 -> tready30/1  "tready_gi1_out"
  GI25/2 -> AXI FIFO26/2  "tvalid_in_FIFO"
  AXI FIFO28/3 -> GI27/3
  AXI FIFO31/3 -> GI30/3
  tdata30/1 -> GI31/1  "tdata_gi1_in"
  AXI FIFO29/3 -> GI28/3
  AXI FIFO30/3 -> GI29/3
  tready_in26/1 -> AXI FIFO27/1  "tready1"
  tready_in31/1 -> AXI FIFO24/1  "tready1"
  tready_in30/1 -> AXI FIFO31/1  "tready1"
  tready_in28/1 -> AXI FIFO29/1  "tready1"
  tdata27/1 -> GI28/1  "tdata_gi1_in"
  GI31/2 -> AXI FIFO24/2  "tvalid_in_FIFO"
  tvalid24/1 -> GI25/2  "tvalid_gi1_in"
  tdata31/1 -> GI32/1  "tdata_gi1_in"
  GI26/1 -> AXI FIFO27/3  "tdata_in_FIFO"
  GI26/3 -> tready25/1  "tready_gi1_out"
  tdata29/1 -> GI30/1  "tdata_gi1_in"
  GI30/3 -> tready29/1  "tready_gi1_out"
  tdata24/1 -> GI25/1  "tdata_gi1_in"
  tready_in25/1 -> AXI FIFO26/1  "tready1"
  tvalid27/1 -> GI28/2  "tvalid_gi1_in"
  tvalid25/1 -> GI26/2  "tvalid_gi1_in"
  GI28/1 -> AXI FIFO29/3  "tdata_in_FIFO"
  tready_in27/1 -> AXI FIFO28/1  "tready1"
  GI27/1 -> AXI FIFO28/3  "tdata_in_FIFO"
  AXI FIFO24/3 -> GI31/3
  AXI FIFO25/3 -> GI32/3
  AXI FIFO27/3 -> GI26/3
  AXI FIFO26/2 -> BitBasher24/1  "tdata_out_FIFO"
  AXI FIFO27/2 -> BitBasher25/1  "tdata_out_FIFO"
  AXI FIFO28/2 -> BitBasher26/1  "tdata_out_FIFO"
  AXI FIFO29/2 -> BitBasher27/1  "tdata_out_FIFO"
  AXI FIFO30/2 -> BitBasher28/1  "tdata_out_FIFO"
  AXI FIFO31/2 -> BitBasher29/1  "tdata_out_FIFO"
  AXI FIFO24/2 -> BitBasher30/1  "tdata_out_FIFO"
  AXI FIFO25/2 -> BitBasher31/1  "tdata_out_FIFO"
  AXI FIFO/1 -> Logical1/1  "tvalid_out_FIFO"
  AXI FIFO1/1 -> Logical1/2  "tvalid_out_FIFO"
  AXI FIFO2/1 -> Logical1/3  "tvalid_out_FIFO"
  AXI FIFO3/1 -> Logical1/4  "tvalid_out_FIFO"
  AXI FIFO4/1 -> Logical1/5  "tvalid_out_FIFO"
  AXI FIFO5/1 -> Logical1/6  "tvalid_out_FIFO"
  AXI FIFO6/1 -> Logical1/7  "tvalid_out_FIFO"
  AXI FIFO7/1 -> Logical1/8  "tvalid_out_FIFO"
  AXI FIFO8/1 -> Logical1/9  "tvalid_out_FIFO"
  AXI FIFO9/1 -> Logical1/10  "tvalid_out_FIFO"
  AXI FIFO10/1 -> Logical1/11  "tvalid_out_FIFO"
  AXI FIFO11/1 -> Logical1/12  "tvalid_out_FIFO"
  AXI FIFO12/1 -> Logical1/13  "tvalid_out_FIFO"
  AXI FIFO13/1 -> Logical1/14
  AXI FIFO16/1 -> Logical1/15  "tvalid_out_FIFO"
  AXI FIFO17/1 -> Logical1/16  "tvalid_out_FIFO"
  AXI FIFO18/1 -> Logical1/17  "tvalid_out_FIFO"
  AXI FIFO19/1 -> Logical1/18  "tvalid_out_FIFO"
  AXI FIFO20/1 -> Logical1/19  "tvalid_out_FIFO"
  AXI FIFO21/1 -> Logical1/20  "tvalid_out_FIFO"
  AXI FIFO22/1 -> Logical1/21  "tvalid_out_FIFO"
  AXI FIFO23/1 -> Logical1/22  "tvalid_out_FIFO"
  AXI FIFO14/1 -> Logical1/23  "tvalid_out_FIFO"
  AXI FIFO15/1 -> Logical1/24  "tvalid_out_FIFO"
  AXI FIFO26/1 -> Logical1/25  "tvalid_out_FIFO"
  AXI FIFO27/1 -> Logical1/26  "tvalid_out_FIFO"
  AXI FIFO28/1 -> Logical1/27  "tvalid_out_FIFO"
  AXI FIFO29/1 -> Logical1/28  "tvalid_out_FIFO"
  AXI FIFO30/1 -> Logical1/29  "tvalid_out_FIFO"
  AXI FIFO31/1 -> Logical1/30  "tvalid_out_FIFO"
  AXI FIFO24/1 -> Logical1/31  "tvalid_out_FIFO"
  AXI FIFO25/1 -> Logical1/32  "tvalid_out_FIFO"
  Vector Delay/1 -> re_out/1

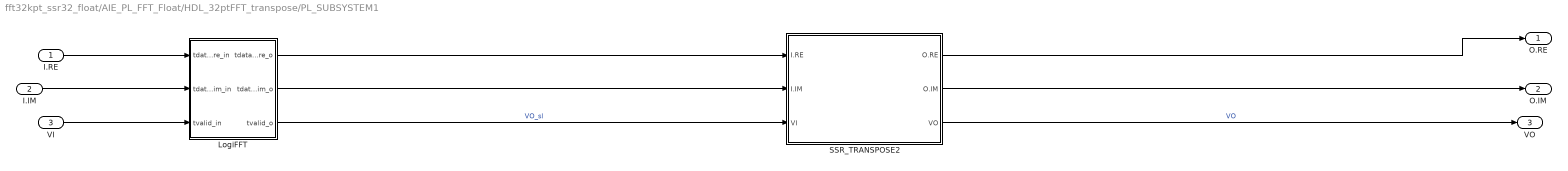
== system fft32kpt_ssr32_float/AIE_PL_FFT_Float/HDL_32ptFFT_transpose/PL_SUBSYSTEM1 ==
  I.RE : Inport
  I.IM : Inport  Port=2
  VI : Inport  Port=3
  LogiFFT : Subsystem
  SSR_TRANSPOSE2 : Subsystem  mask{SSR=SSR, MEM_STYLE=0, M=M, N=N1, DATA_WIDTH=DATA_WIDTH}
      mask prompts: MEM_STYLE "Memory Style"
  O.RE : Outport
  O.IM : Outport  Port=2
  VO : Outport  Port=3
  wires:
  I.RE/1 -> LogiFFT/1(tdata_re_in)
  I.IM/1 -> LogiFFT/2(tdata_im_in)
  LogiFFT/1(tdata_re_o) -> SSR_TRANSPOSE2/1("I.RE ")
  VI/1 -> LogiFFT/3(tvalid_in)
  SSR_TRANSPOSE2/1(" O.RE") -> O.RE/1
  SSR_TRANSPOSE2/2(" O.IM") -> O.IM/1
  SSR_TRANSPOSE2/3(" VO") -> VO/1  "VO"
  LogiFFT/2(tdata_im_o) -> SSR_TRANSPOSE2/2("I.IM ")
  LogiFFT/3(tvalid_o) -> SSR_TRANSPOSE2/3("VI ")  "VO_sl"
